simulink model "prelim_control_sys"  (R2016a)
settings: Solver=VariableStepAuto  StartTime=0.0  StopTime=10.0  RelTol=1e-3
values from neighbouring files (symbols this model uses):
  Kr = -inv(Cd*inv(Ad-eye(n)-Bd*K)*Bd)    [SSE_sim.m]    (also in SSE_sim_md.m)
settings Model: Creator=rcyprus  LastModifiedBy=rcyprus

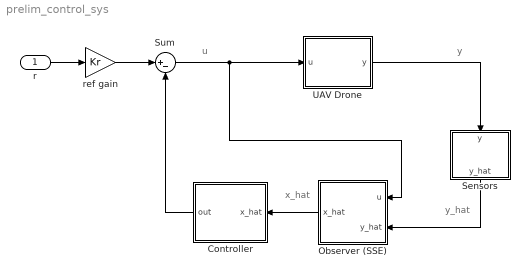
== system prelim_control_sys ==
  note: u
  note: y_hat
  note: y
  note: x_hat
  r : Inport
  Controller : Subsystem
  Observer (SSE) : Subsystem
  Sensors : Subsystem
  Sum : Sum  Inputs=|+-
  UAV Drone : Subsystem
  ref gain : Gain  Gain=Kr
  wires:
  ref gain/1 -> Sum/1
  r/1 -> ref gain/1
  Sum/1 -> UAV Drone/1(u), Observer (SSE)/1(u)
  Controller/1(out) -> Sum/2
  Observer (SSE)/1(x_hat) -> Controller/1(x_hat)
  Sensors/1(y_hat) -> Observer (SSE)/2(y_hat)
  UAV Drone/1(y) -> Sensors/1(y)

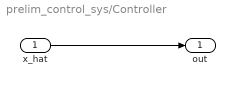
== system prelim_control_sys/Controller ==
  x_hat : Inport
  out : Outport
  wires:
  x_hat/1 -> out/1

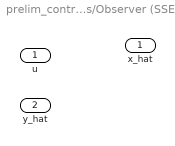
== system prelim_control_sys/Observer (SSE) ==
  u : Inport
  y_hat : Inport  Port=2
  x_hat : Outport

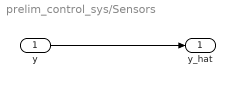
== system prelim_control_sys/Sensors ==
  y : Inport
  y_hat : Outport
  wires:
  y/1 -> y_hat/1

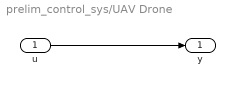
== system prelim_control_sys/UAV Drone ==
  u : Inport
  y : Outport
  wires:
  u/1 -> y/1
